simulink model "Simulink Model AC-DC Power Transmission"  (R2024a)
settings: Solver=VariableStepAuto  StartTime=0.0  StopTime=5  RelTol=1e-3
values from neighbouring files (symbols this model uses):
  C1 = 1e-3    (= 0.001)    [Parameters.m]
  Ka = Vdcref/2    [Parameters.m]
  kii1 = 2*3.14*fbwi*R1/Ka    [Parameters.m]
  kiw1 = kpw1/a1^2/taul1    [Parameters.m]
  kpi1 = 2*3.14*fbwi*L1/Ka    [Parameters.m]
  kpw1 = 2*C1/k1/a1/taul1    [Parameters.m]
  L1 = 5e-3    (= 0.005)    [Parameters.m]
  m = 0.848    [Parameters.m]
  R1 = 0.001    [Parameters.m]
  Rbat = (Vdcref/Pdc)*(Vbat-Vdcref)    [Parameters.m]
  tauf1 = 1/2/3.14/100    (= 0.0015923566879)    [Parameters.m]
  Vbat = 900    [Parameters.m]
  Vdcref = 400*sqrt(2)*2/(m*sqrt(3))    [Parameters.m]
  Vll = 400    [Parameters.m]
  w = 2*pi*f    (= 314.159265359)    [Parameters.m]
libraries: spsSeriesRLCBranchLib x9, spsIGBTDiodeLib x6, spsVoltageMeasurementLib x3, spsCurrentMeasurementLib x3, spsBreakerLib x1, spsDCVoltageSourceLib x1, spsTriangleGeneratorLib x1, spsThreePhaseBreakerLib x1, spsThreePhaseSourceLib x1, sps_lib x1
settings Model: SimulationMode=accelerator  Creator=akash  LastModifiedBy=Rhythm Shah
settings SolverCC: ZeroCrossAlgorithm=Adaptive
settings DebuggingCC: IgnoredZcDiagnostic=none

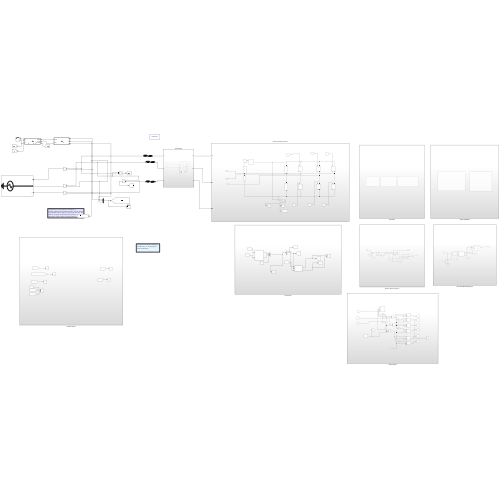
[thumbnail: Simulink's stored preview of the top-level diagram]
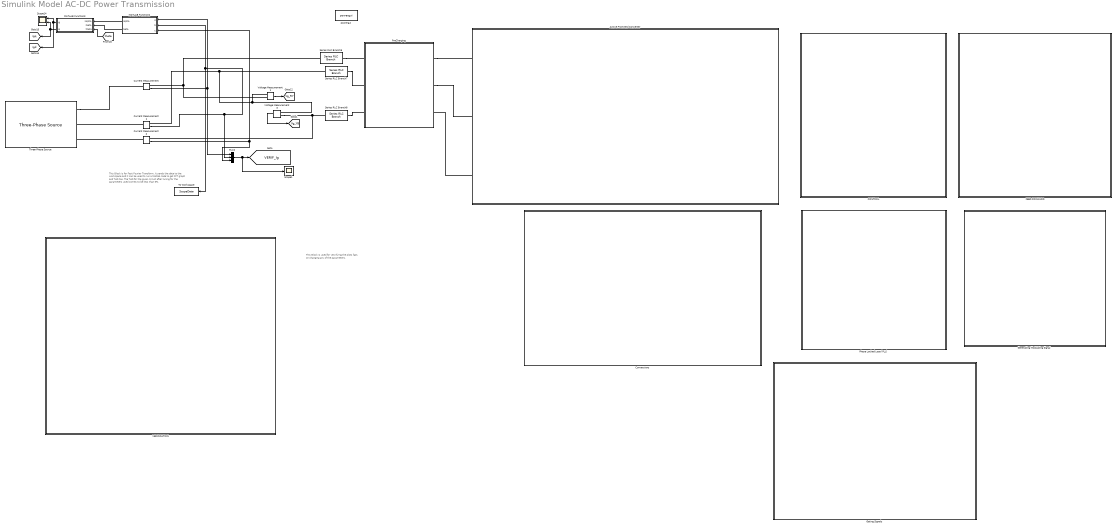
== system Simulink Model AC-DC Power Transmission ==
  note: This Block is used for veryifying
      | the plots fast, on changing any
      | of the parameters.
  note: This Block is for Fast Fourier Transform, it
      | sends the data to the workspace and it can be used to
      | run a Matlab code to get FFT graph and THD too. The
      | THD for the given circuit after tuning for the
      | parameters used comes to be less than 5%.
  Active Front End Converter : Subsystem
  CONTROL : Subsystem
  Conversions : Subsystem
  Current Measurement : spsCurrentMeasurementLib/Current Measurement  PhasorSimulation=off  OutputType=Complex  PSBequivalent=0
  Current Measurement1 : spsCurrentMeasurementLib/Current Measurement  PhasorSimulation=off  OutputType=Complex  PSBequivalent=0
  Current Measurement2 : spsCurrentMeasurementLib/Current Measurement  PhasorSimulation=off  OutputType=Complex  PSBequivalent=0
  FEED FORWARD : Subsystem
  Gating Signals : Subsystem
  Generating Modulating Signal : Subsystem
  MATLAB Function2 : MATLAB Function  TreatAsAtomicUnit=on
  MATLAB Function3 : MATLAB Function  TreatAsAtomicUnit=on
  Mux2 : Mux  Inputs=3
  Phase Locked Loop (PLL) : Subsystem
  PreCharging : Subsystem
  Scope1 : Scope
  Scope14 : Scope  NumInputPorts=2
  Series RLC Branch6 : spsSeriesRLCBranchLib/Series RLC Branch  LConnTagsString=__new0  RConnTagsString=__new0  BranchType=RL  Resistance=R1  Inductance=L1  SetiL0=off  InitialCurrent=0  Capacitance=1e-6  Setx0=off  InitialVoltage=0  Measurements=None
  Series RLC Branch7 : spsSeriesRLCBranchLib/Series RLC Branch  LConnTagsString=__new0  RConnTagsString=__new0  BranchType=RL  Resistance=R1  Inductance=L1  SetiL0=off  InitialCurrent=0  Capacitance=1e-6  Setx0=off  InitialVoltage=0  Measurements=None
  Series RLC Branch8 : spsSeriesRLCBranchLib/Series RLC Branch  LConnTagsString=__new0  RConnTagsString=__new0  BranchType=RL  Resistance=R1  Inductance=L1  SetiL0=off  InitialCurrent=0  Capacitance=1e-6  Setx0=off  InitialVoltage=0  Measurements=None
  Three-Phase Source : spsThreePhaseSourceLib/Three-Phase Source  InternalConnection=Yg  VoltagePhases=off  Voltage=Vll  PhaseAngle=0  Voltage_phases=[25e3 25e3 25e3]/sqrt(3)  PhaseAngles_phases=[0 -120 +120]  Frequency=50  NonIdealSource=off  SpecifyImpedance=off  Resistance=0  Inductance=0  ShortCircuitLevel=100e6  BaseVoltage=0  XRratio=7  BusType=swing  Pref=10e3  Qref=0  Prefabc=[10e3, 10e3, 10e3]  Qrefabc=[0, 0, 0]  Qmin=-inf  Qmax=inf
  To Workspace : ToWorkspace  VariableName=ScopeData  SaveFormat=Structure With Time  SampleTime=-1
  VERIFICATION : Subsystem
  Voltage Measurement1 : spsVoltageMeasurementLib/Voltage Measurement  PhasorSimulation=off  OutputType=Complex  PSBequivalent=0
  Voltage Measurement3 : spsVoltageMeasurementLib/Voltage Measurement  PhasorSimulation=off  OutputType=Complex  PSBequivalent=0
  powergui : sps_lib/powergui  Priority=1  SimulationMode=Continuous  SampleTime=50e-6  frequency=60  Iterations=50  frequencyindice=0  Pbase=100e6  ErrMax=1e-4  UnitsV=kV  UnitsW=MW  buscounter=0  FunctionMessages=off  echomessages=off  EnableUseOfTLC=off  CurrentSourceSwitches=off  DisableSnubberDevices=off  DisableRonSwitches=off  DisableVfSwitches=off  DisplayEquations=off  AutomaticDiscreteSolvers=off  SolverType=Tustin/Backward Euler (TBE)  Interpol=off  ExternalGateDelay=off  methode=off  Ts=100  x0status=blocks  SPID=on  SwTol=0  HookPort=off  NonlinearTolerance=1e-4  nMaxIteration=100  ContinueOnMaxIteration=off  RestoreLinks=warning  ResistiveCurrentMeasurement=off  Frange=[0:2:500]  Ylog=off  Xlog=on  ShowGrid=off  save=off  variable=ZData  structure=0  ZoomFFT=off  StartTime=0.0  cycles=1  DisplayStyle=1  fundamental=60  FreqAxis=off  MaxFrequency=1000  frequencyindicesteady=1  RmsSteady=1  display=off
  tag scope: VERIF_Ig=global, Vg_RY=global, Vg_YB=global, igd=global, igq=global
  wires:
  Current Measurement1/1 -> MATLAB Function2/2(b), To Workspace/1, Mux2/2
  Current Measurement/1 -> Mux2/1, MATLAB Function2/1(a)
  Current Measurement2/1 -> MATLAB Function2/3(c), Mux2/3
  Voltage Measurement1/1 -> [Vg_RY]
  Voltage Measurement3/1 -> [Vg_YB]
  Mux2/1 -> [VERIF_Ig], Scope1/1
  MATLAB Function3/2(iq) -> [igq], Scope14/2
  [theta] -> MATLAB Function3/3(theta)
  MATLAB Function2/2(beta) -> MATLAB Function3/2(ibeta)
  MATLAB Function2/1(alpha) -> MATLAB Function3/1(ialpha)
  MATLAB Function3/1(id) -> [igd], Scope14/1
  connections:
  Voltage Measurement3/LConn2 -- Current Measurement2/RConn1 -- Series RLC Branch8/RConn1
  Voltage Measurement1/LConn2 -- Current Measurement1/RConn1 -- Series RLC Branch7/RConn1 -- Voltage Measurement3/LConn1
  Voltage Measurement1/LConn1 -- Current Measurement/RConn1 -- Series RLC Branch6/RConn1
  Three-Phase Source/RConn1 -- Current Measurement/LConn1
  Current Measurement2/LConn1 -- Three-Phase Source/RConn3
  Current Measurement1/LConn1 -- Three-Phase Source/RConn2
  PreCharging/LConn1 -- Active Front End Converter/RConn1
  PreCharging/LConn2 -- Active Front End Converter/RConn2
  Series RLC Branch6/LConn1 -- PreCharging/RConn1
  Series RLC Branch7/LConn1 -- PreCharging/RConn2
  Active Front End Converter/RConn3 -- PreCharging/LConn3
  Series RLC Branch8/LConn1 -- PreCharging/RConn3

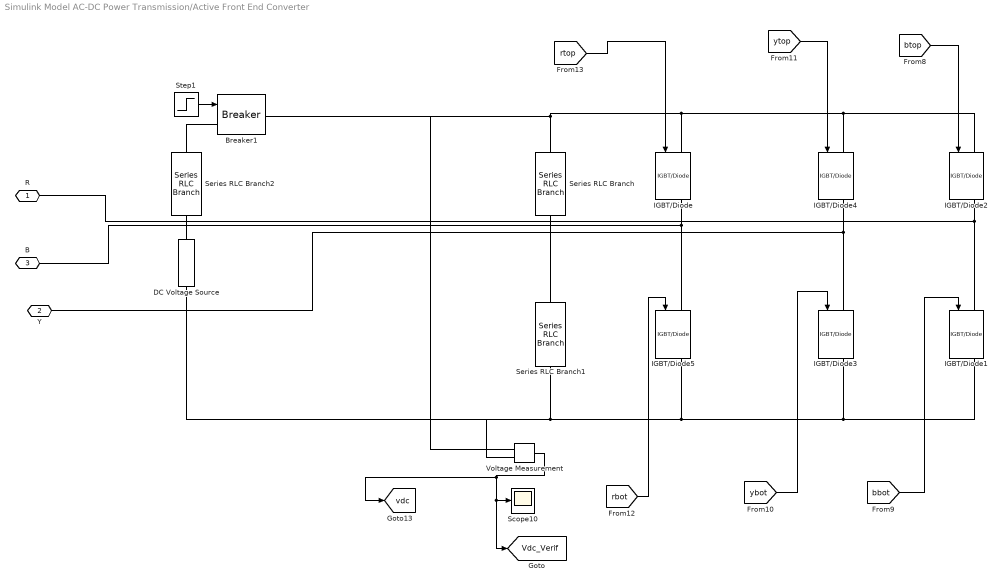
== system Simulink Model AC-DC Power Transmission/Active Front End Converter ==
  Breaker1 : spsBreakerLib/Breaker  InitialState=0  SwitchingTimes="[1/60  5/60]"  External=on  BreakerResistance=0.01  SnubberResistance=1e6  SnubberCapacitance=inf  Measurements=None  MoreParameters=on  NoBreakLoop=off
  DC Voltage Source : spsDCVoltageSourceLib/DC Voltage Source  Amplitude=Vbat  Measurements=None
  IGBT/Diode{,1..5} (6 alike) : spsIGBTDiodeLib/IGBT//Diode  Ron=1e-5  Rs=1e7  Cs=inf  Measurements=on
  Scope10 : Scope
  Series RLC Branch : spsSeriesRLCBranchLib/Series RLC Branch  LConnTagsString=__new0  RConnTagsString=__new0  BranchType=C  Resistance=0  Inductance=0  SetiL0=off  InitialCurrent=0  Capacitance=C1  Setx0=on  InitialVoltage=0  Measurements=None
  Series RLC Branch1 : spsSeriesRLCBranchLib/Series RLC Branch  LConnTagsString=__new0  RConnTagsString=__new0  BranchType=C  Resistance=0  Inductance=0  SetiL0=off  InitialCurrent=0  Capacitance=C1  Setx0=on  InitialVoltage=0  Measurements=None
  Series RLC Branch2 : spsSeriesRLCBranchLib/Series RLC Branch  LConnTagsString=__new0  RConnTagsString=__new0  BranchType=R  Resistance=Rbat  Inductance=0  SetiL0=off  InitialCurrent=0  Capacitance=1e-6  Setx0=off  InitialVoltage=0  Measurements=None
  Step1 : Step  Time=0.6  SampleTime=0
  Voltage Measurement : spsVoltageMeasurementLib/Voltage Measurement  PhasorSimulation=off  OutputType=Complex  PSBequivalent=0
  R : PMIOPort  Side=Right
  Y : PMIOPort  Port=2  Side=Right
  B : PMIOPort  Port=3  Side=Right
  tag scope: Vdc_Verif=global, vdc=global
  wires:
  [ybot] -> IGBT/Diode3/1
  [rtop] -> IGBT/Diode/1
  [bbot] -> IGBT/Diode1/1
  [ytop] -> IGBT/Diode4/1
  Step1/1 -> Breaker1/1
  [rbot] -> IGBT/Diode5/1
  [btop] -> IGBT/Diode2/1
  Voltage Measurement/1 -> [vdc], [Vdc_Verif], Scope10/1
  connections:
  IGBT/Diode4/RConn1 -- IGBT/Diode3/LConn1 -- Y/RConn1
  IGBT/Diode2/RConn1 -- IGBT/Diode1/LConn1 -- R/RConn1
  Breaker1/LConn1 -- Series RLC Branch2/LConn1
  IGBT/Diode3/RConn1 -- Series RLC Branch1/RConn1 -- DC Voltage Source/LConn1 -- Voltage Measurement/LConn2 -- IGBT/Diode5/RConn1 -- IGBT/Diode1/RConn1
  IGBT/Diode4/LConn1 -- IGBT/Diode/LConn1 -- Voltage Measurement/LConn1 -- Breaker1/RConn1 -- Series RLC Branch/LConn1 -- IGBT/Diode2/LConn1
  IGBT/Diode/RConn1 -- B/RConn1 -- IGBT/Diode5/LConn1
  DC Voltage Source/RConn1 -- Series RLC Branch2/RConn1
  Series RLC Branch1/LConn1 -- Series RLC Branch/RConn1

== system Simulink Model AC-DC Power Transmission/CONTROL ==
  Id Current control : Subsystem
  Iq Current Control : Subsystem
  Voltage control : Subsystem

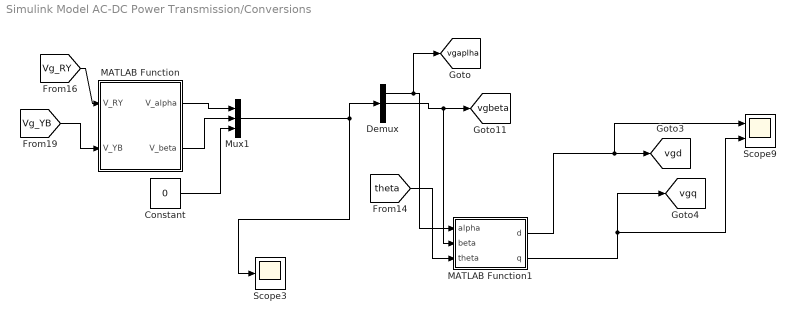
== system Simulink Model AC-DC Power Transmission/Conversions ==
  Constant : Constant  Value=0
  Demux : Demux  Outputs=3
  MATLAB Function : MATLAB Function  TreatAsAtomicUnit=on
  MATLAB Function1 : MATLAB Function  TreatAsAtomicUnit=on
  Mux1 : Mux  Inputs=3
  Scope3 : Scope
  Scope9 : Scope  NumInputPorts=2
  tag scope: vgaplha=global, vgbeta=global, vgd=global, vgq=global
  wires:
  Mux1/1 -> Scope3/1, Demux/1
  MATLAB Function/1(V_alpha) -> Mux1/1
  Demux/2 -> MATLAB Function1/2(beta), [vgbeta]
  Demux/1 -> MATLAB Function1/1(alpha), [vgaplha]
  MATLAB Function1/2(q) -> [vgq], Scope9/2
  [Vg_YB] -> MATLAB Function/2(V_YB)
  MATLAB Function1/1(d) -> Scope9/1, [vgd]
  [theta] -> MATLAB Function1/3(theta)
  MATLAB Function/2(V_beta) -> Mux1/2
  [Vg_RY] -> MATLAB Function/1(V_RY)
  Constant/1 -> Mux1/3

== system Simulink Model AC-DC Power Transmission/FEED FORWARD ==
  Id Feed Forward : Subsystem
  Iq Feed Forward : Subsystem

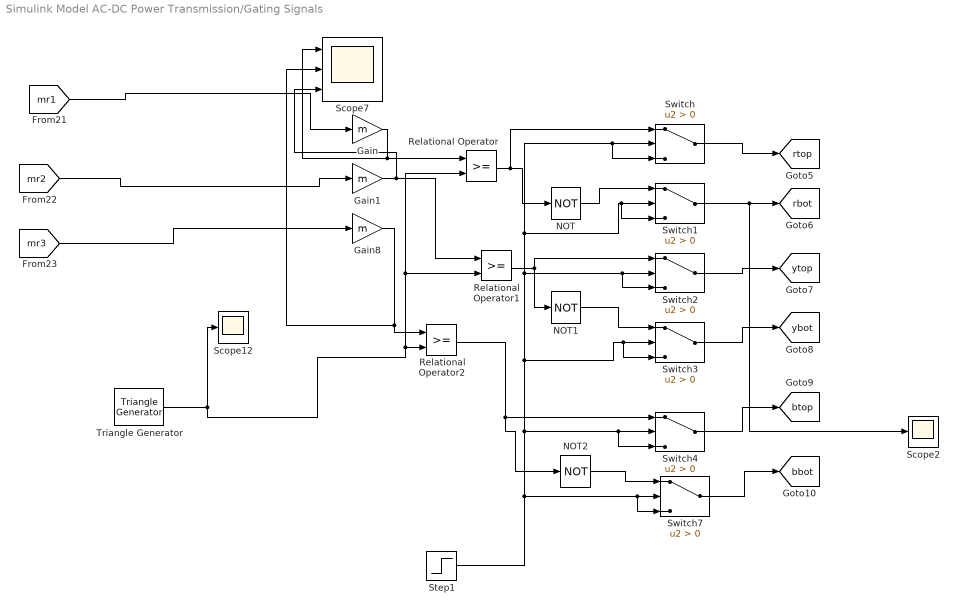
== system Simulink Model AC-DC Power Transmission/Gating Signals ==
  Gain : Gain  Gain=m
  Gain1 : Gain  Gain=m
  Gain8 : Gain  Gain=m
  NOT : Logic  Operator=NOT  IconShape=distinctive  AllPortsSameDT=off  OutDataTypeStr=boolean
  NOT1 : Logic  Operator=NOT  IconShape=distinctive  AllPortsSameDT=off  OutDataTypeStr=boolean
  NOT2 : Logic  Operator=NOT  IconShape=distinctive  AllPortsSameDT=off  OutDataTypeStr=boolean
  Relational Operator : RelationalOperator  OutDataTypeStr=boolean  RndMeth=Simplest  InputSameDT=off
  Relational Operator1 : RelationalOperator  OutDataTypeStr=boolean  RndMeth=Simplest  InputSameDT=off
  Relational Operator2 : RelationalOperator  OutDataTypeStr=boolean  RndMeth=Simplest  InputSameDT=off
  Scope12 : Scope
  Scope2 : Scope
  Scope7 : Scope  NumInputPorts=3
  Step1 : Step  SampleTime=0
  Switch{,1..4,7} (6 alike) : Switch  Criteria=u2 > Threshold  SaturateOnIntegerOverflow=off  InputSameDT=off
  Triangle Generator : spsTriangleGeneratorLib/Triangle Generator  Freq=5000  Phase=0  Ts=0
  tag scope: bbot=global, btop=global, rbot=global, rtop=global, ybot=global, ytop=global
  wires:
  NOT/1 -> Switch1/1
  [mr3] -> Gain8/1
  Switch1/1 -> Scope2/1, [rbot]
  Gain1/1 -> Relational Operator1/1, Scope7/3
  Gain/1 -> Relational Operator/1, Scope7/1
  Switch7/1 -> [bbot]
  NOT2/1 -> Switch7/1
  Triangle Generator/1 -> Relational Operator2/2, Relational Operator1/2, Relational Operator/2, Scope12/1
  Relational Operator1/1 -> Switch2/1, NOT1/1
  Relational Operator/1 -> Switch/1, NOT/1
  [mr1] -> Gain/1
  Switch2/1 -> [ytop]
  Step1/1 -> Switch7/3, Switch7/2, Switch4/3, Switch4/2, Switch3/3, Switch3/2, Switch1/3, Switch1/2, Switch/3, Switch/2, Switch2/3, Switch2/2
  Gain8/1 -> Scope7/2, Relational Operator2/1
  Relational Operator2/1 -> NOT2/1, Switch4/1
  [mr2] -> Gain1/1
  Switch3/1 -> [ybot]
  Switch/1 -> [rtop]
  Switch4/1 -> [btop]
  NOT1/1 -> Switch3/1

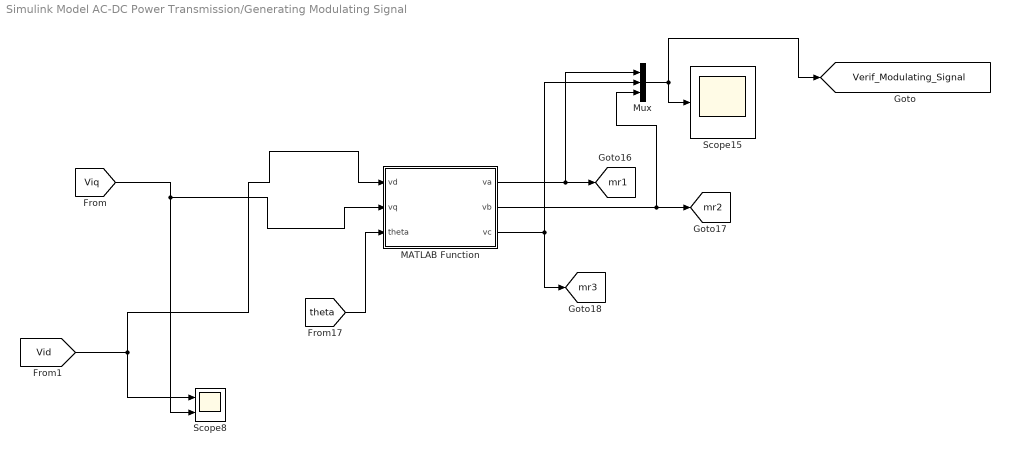
== system Simulink Model AC-DC Power Transmission/Generating Modulating Signal ==
  MATLAB Function : MATLAB Function  TreatAsAtomicUnit=on
  Mux : Mux  Inputs=3
  Scope15 : Scope
  Scope8 : Scope  NumInputPorts=2
  tag scope: Verif_Modulating_Signal=global, mr1=global, mr2=global, mr3=global
  wires:
  MATLAB Function/1(va) -> Mux/1, [mr1]
  MATLAB Function/2(vb) -> Mux/3, [mr2]
  [theta] -> MATLAB Function/3(theta)
  [Vid] -> MATLAB Function/1(vd), Scope8/1
  MATLAB Function/3(vc) -> Mux/2, [mr3]
  [Viq] -> Scope8/2, MATLAB Function/2(vq)
  Mux/1 -> [Verif_Modulating_Signal], Scope15/1

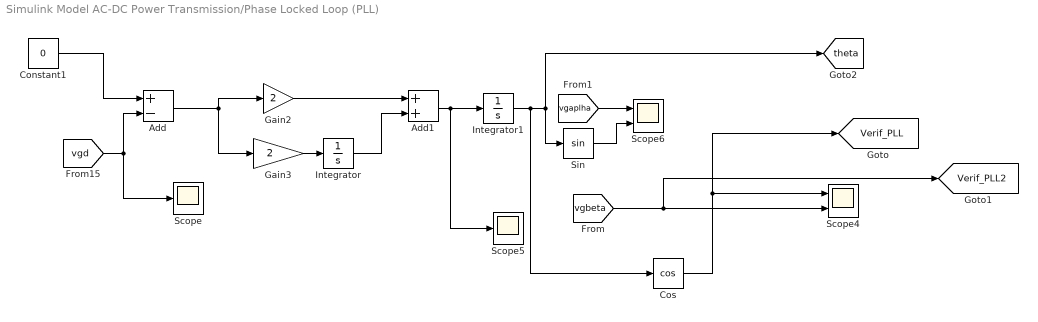
== system Simulink Model AC-DC Power Transmission/Phase Locked Loop (PLL) ==
  Add : Sum  Inputs=+-
  Add1 : Sum
  Constant1 : Constant  Value=0
  Cos : Trigonometry  Operator=cos
  Gain2 : Gain  Gain=2
  Gain3 : Gain  Gain=2
  Integrator : Integrator
  Integrator1 : Integrator
  Scope : Scope
  Scope4 : Scope  NumInputPorts=2
  Scope5 : Scope
  Scope6 : Scope  NumInputPorts=2
  Sin : Trigonometry
  tag scope: Verif_PLL2=global, Verif_PLL=global, theta=global
  wires:
  Constant1/1 -> Add/1
  [vgbeta] -> [Verif_PLL2], Scope4/2
  Integrator/1 -> Add1/2
  Gain3/1 -> Integrator/1
  [vgd] -> Scope/1, Add/2
  Sin/1 -> Scope6/2
  Gain2/1 -> Add1/1
  Integrator1/1 -> Cos/1, [theta], Sin/1
  Add/1 -> Gain3/1, Gain2/1
  Add1/1 -> Scope5/1, Integrator1/1
  Cos/1 -> [Verif_PLL], Scope4/1
  [vgaplha] -> Scope6/1

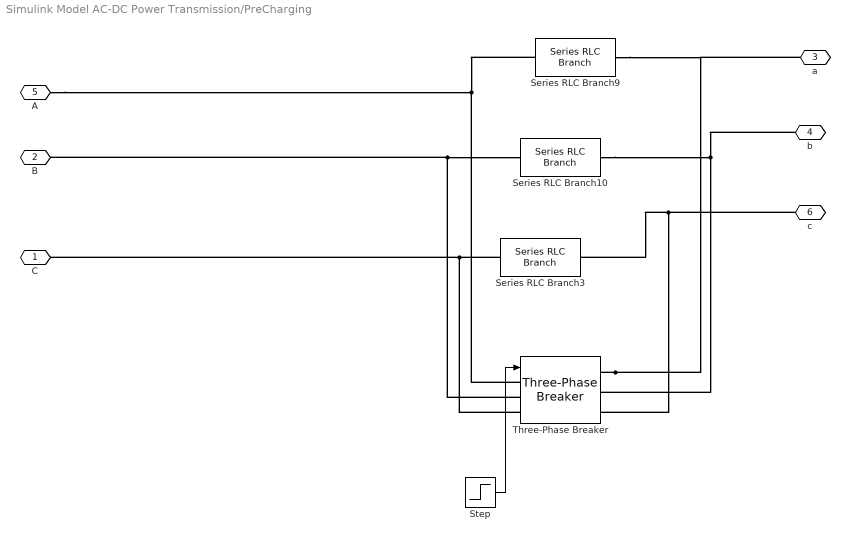
== system Simulink Model AC-DC Power Transmission/PreCharging ==
  Series RLC Branch10 : spsSeriesRLCBranchLib/Series RLC Branch  LConnTagsString=__new0  RConnTagsString=__new0  BranchType=R  Resistance=50  Inductance=1e-3  SetiL0=off  InitialCurrent=0  Capacitance=1e-6  Setx0=off  InitialVoltage=0  Measurements=None
  Series RLC Branch3 : spsSeriesRLCBranchLib/Series RLC Branch  LConnTagsString=__new0  RConnTagsString=__new0  BranchType=R  Resistance=50  Inductance=1e-3  SetiL0=off  InitialCurrent=0  Capacitance=1e-6  Setx0=off  InitialVoltage=0  Measurements=None
  Series RLC Branch9 : spsSeriesRLCBranchLib/Series RLC Branch  LConnTagsString=__new0  RConnTagsString=__new0  BranchType=R  Resistance=50  Inductance=1e-3  SetiL0=off  InitialCurrent=0  Capacitance=1e-6  Setx0=off  InitialVoltage=0  Measurements=None
  Step : Step  Time=0.6  SampleTime=0
  Three-Phase Breaker : spsThreePhaseBreakerLib/Three-Phase Breaker  InitialState=open  SwitchA=on  SwitchB=on  SwitchC=on  SwitchTimes="[1/60  5/60]"  External=on  BreakerResistance=0.01  SnubberResistance=1e6  SnubberCapacitance=inf  Measurements=None
  C : PMIOPort  Side=Left
  B : PMIOPort  Port=2  Side=Left
  a : PMIOPort  Port=3  Side=Right
  b : PMIOPort  Port=4  Side=Right
  A : PMIOPort  Port=5  Side=Left
  c : PMIOPort  Port=6  Side=Right
  wires:
  Step/1 -> Three-Phase Breaker/1
  connections:
  Three-Phase Breaker/RConn1 -- a/RConn1 -- Series RLC Branch9/RConn1
  c/RConn1 -- Three-Phase Breaker/RConn3 -- Series RLC Branch3/RConn1
  Three-Phase Breaker/LConn3 -- C/RConn1 -- Series RLC Branch3/LConn1
  Series RLC Branch10/RConn1 -- b/RConn1 -- Three-Phase Breaker/RConn2
  Three-Phase Breaker/LConn2 -- Series RLC Branch10/LConn1 -- B/RConn1
  Series RLC Branch9/LConn1 -- Three-Phase Breaker/LConn1 -- A/RConn1

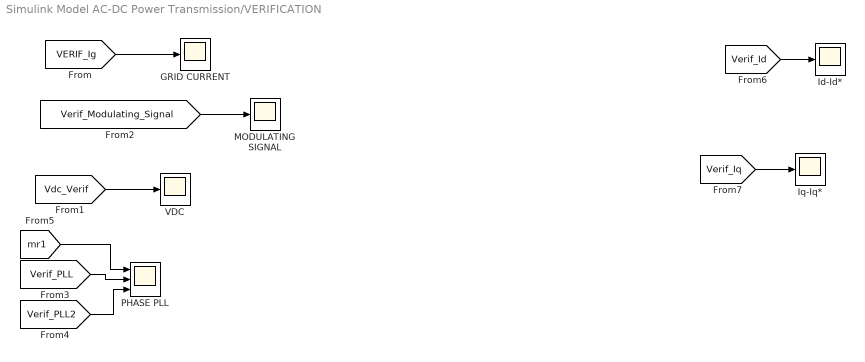
== system Simulink Model AC-DC Power Transmission/VERIFICATION ==
  GRID CURRENT : Scope
  Id-Id* : Scope
  Iq-Iq* : Scope
  MODULATING SIGNAL : Scope
  PHASE PLL : Scope  NumInputPorts=3
  VDC : Scope
  wires:
  [VERIF_Ig] -> GRID CURRENT/1
  [Verif_Modulating_Signal] -> MODULATING SIGNAL/1
  [Vdc_Verif] -> VDC/1
  [Verif_PLL] -> PHASE PLL/2
  [Verif_PLL2] -> PHASE PLL/3
  [mr1] -> PHASE PLL/1
  [Verif_Id] -> Id-Id*/1
  [Verif_Iq] -> Iq-Iq*/1

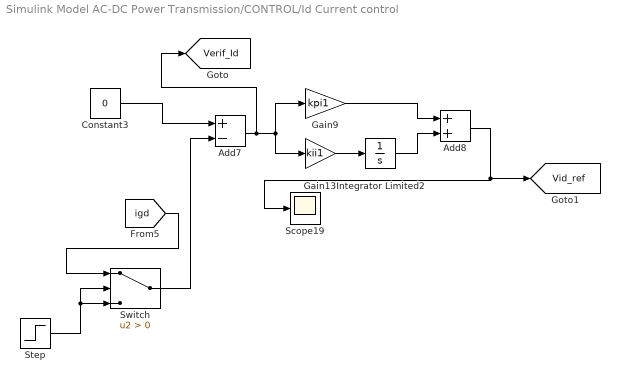
== system Simulink Model AC-DC Power Transmission/CONTROL/Id Current control ==
  Add7 : Sum  Inputs=+-
  Add8 : Sum
  Constant3 : Constant  Value=0
  Gain13 : Gain  Gain=kii1
  Gain9 : Gain  Gain=kpi1
  Integrator Limited2 : Integrator  LimitOutput=on  UpperSaturationLimit=1  LowerSaturationLimit=-1
  Scope19 : Scope
  Step : Step  SampleTime=0
  Switch : Switch  Criteria=u2 > Threshold  SaturateOnIntegerOverflow=off  InputSameDT=off
  tag scope: Verif_Id=global, Vid_ref=global
  wires:
  Gain13/1 -> Integrator Limited2/1
  Integrator Limited2/1 -> Add8/2
  Constant3/1 -> Add7/1
  Gain9/1 -> Add8/1
  Add7/1 -> [Verif_Id], Gain9/1, Gain13/1
  Add8/1 -> Scope19/1, [Vid_ref]
  Step/1 -> Switch/3, Switch/2
  Switch/1 -> Add7/2
  [igd] -> Switch/1

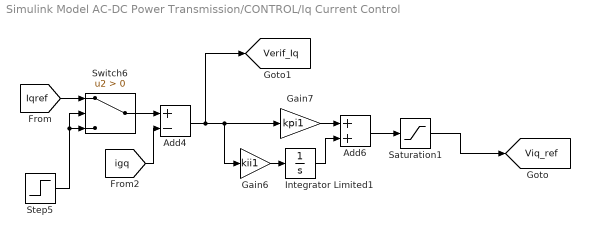
== system Simulink Model AC-DC Power Transmission/CONTROL/Iq Current Control ==
  Add4 : Sum  Inputs=+-
  Add6 : Sum
  Gain6 : Gain  Gain=kii1
  Gain7 : Gain  Gain=kpi1
  Integrator Limited1 : Integrator  LimitOutput=on  UpperSaturationLimit=1  LowerSaturationLimit=-1
  Saturation1 : Saturate  UpperLimit=1  LowerLimit=-1
  Step5 : Step  SampleTime=0
  Switch6 : Switch  Criteria=u2 > Threshold  SaturateOnIntegerOverflow=off  InputSameDT=off
  tag scope: Verif_Iq=global, Viq_ref=global
  wires:
  Step5/1 -> Switch6/3, Switch6/2
  Integrator Limited1/1 -> Add6/2
  [igq] -> Add4/2
  Gain7/1 -> Add6/1
  Add4/1 -> [Verif_Iq], Gain6/1, Gain7/1
  Switch6/1 -> Add4/1
  Add6/1 -> Saturation1/1
  Gain6/1 -> Integrator Limited1/1
  [Iqref] -> Switch6/1
  Saturation1/1 -> [Viq_ref]

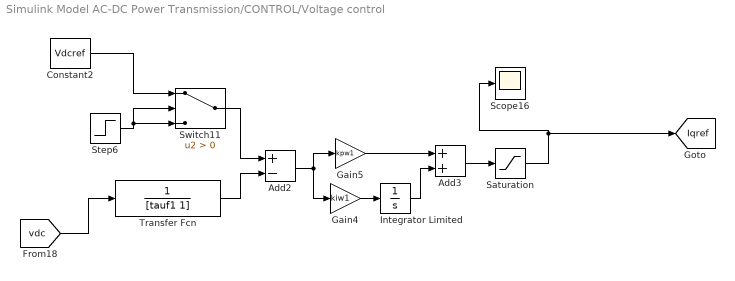
== system Simulink Model AC-DC Power Transmission/CONTROL/Voltage control ==
  Add2 : Sum  Inputs=+-
  Add3 : Sum
  Constant2 : Constant  Value=Vdcref
  Gain4 : Gain  Gain=kiw1
  Gain5 : Gain  Gain=kpw1
  Integrator Limited : Integrator  LimitOutput=on  UpperSaturationLimit=25  LowerSaturationLimit=-25
  Saturation : Saturate  UpperLimit=25  LowerLimit=-25
  Scope16 : Scope
  Step6 : Step  Time=1.5  SampleTime=0
  Switch11 : Switch  Criteria=u2 > Threshold  SaturateOnIntegerOverflow=off  InputSameDT=off
  Transfer Fcn : TransferFcn  Denominator=[tauf1 1]
  tag scope: Iqref=global
  wires:
  Transfer Fcn/1 -> Add2/2
  Integrator Limited/1 -> Add3/2
  Switch11/1 -> Add2/1
  Gain4/1 -> Integrator Limited/1
  [vdc] -> Transfer Fcn/1
  Constant2/1 -> Switch11/1
  Gain5/1 -> Add3/1
  Step6/1 -> Switch11/2, Switch11/3
  Add3/1 -> Saturation/1
  Add2/1 -> Gain4/1, Gain5/1
  Saturation/1 -> [Iqref], Scope16/1

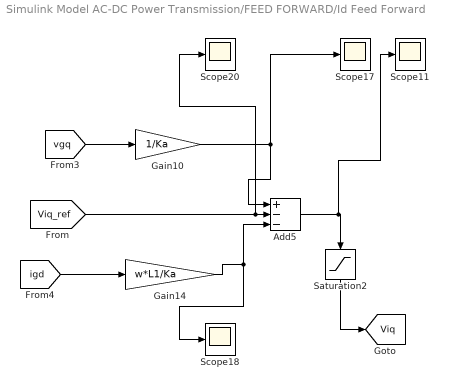
== system Simulink Model AC-DC Power Transmission/FEED FORWARD/Id Feed Forward ==
  Add5 : Sum  Inputs=+--
  Gain10 : Gain  Gain=1/Ka
  Gain14 : Gain  Gain=w*L1/Ka
  Saturation2 : Saturate  UpperLimit=1  LowerLimit=-1
  Scope{11,17..18,20} (4 alike) : Scope
  tag scope: Viq=global
  wires:
  [vgq] -> Gain10/1
  Add5/1 -> Scope11/1, Saturation2/1
  [Viq_ref] -> Scope20/1, Add5/2
  Gain14/1 -> Scope18/1, Add5/3
  [igd] -> Gain14/1
  Saturation2/1 -> [Viq]
  Gain10/1 -> Add5/1, Scope17/1

== system Simulink Model AC-DC Power Transmission/FEED FORWARD/Iq Feed Forward ==
  Add9 : Sum  Inputs=+-+
  Gain11 : Gain  Gain=1/Ka
  Gain12 : Gain  Gain=w*L1/Ka
  Saturation3 : Saturate  UpperLimit=1  LowerLimit=-1
  tag scope: Vid=global
  wires:
  Gain12/1 -> Add9/3
  Saturation3/1 -> [Vid]
  [Vid_ref] -> Add9/2
  [vgd] -> Gain11/1
  Gain11/1 -> Add9/1
  Add9/1 -> Saturation3/1
  [igq] -> Gain12/1

== matlab function Simulink Model AC-DC Power Transmission/Conversions/MATLAB Function1 ==
  data: alpha input; d output; beta input; theta input; q output
function[d,q]=alphabeta_to_dq(alpha, beta, theta)

    d=alpha*cos(theta)+beta*sin(theta);
    q=-alpha*sin(theta)+beta*cos(theta);
end

== matlab function Simulink Model AC-DC Power Transmission/Conversions/MATLAB Function ==
  data: V_RY input; V_alpha output; V_YB input; V_beta output
function [V_alpha , V_beta] = fcn(V_RY,V_YB)
% Convert line-to-line voltages to phase voltages
    V_R = V_RY / sqrt(3) * exp(-1i * pi / 6); % -30 degrees phase shift
    V_Y = V_YB / sqrt(3) * exp(-1i * pi / 6); % -30 degrees phase shift
    
    % Assume balanced system, so V_B = -(V_R + V_Y)
    V_B = -(V_R + V_Y);
    
    % Extract real parts for Clarke Transformation (phase voltages)
    V_R = real(V_R);
    V_Y = real(V_Y);
    V_B = real(V_B);
    
    % Apply Clarke Transform to get alpha-beta components
    V_alph = (2/3) * (V_R - 0.5 * V_Y - 0.5 * V_B);
    V_bet = (2/3) * (sqrt(3)/2 * (V_Y - V_B));
V_alpha = V_alph;
V_beta = V_bet;
end

== matlab function Simulink Model AC-DC Power Transmission/MATLAB Function2 ==
  data: a input; alpha output; b input; c input; beta output
function [alpha,beta]=abctoalphabeta(a,b,c)

    alpha=(2/3)*(a-0.5*b-0.5*c);
    beta=(2/3)*(sqrt(3)/2*(b-c));
end

== matlab function Simulink Model AC-DC Power Transmission/MATLAB Function3 ==
  data: ialpha input; id output; ibeta input; theta input; iq output
function [id,iq]=alphabeta_to_dq(ialpha,ibeta,theta)
    
    id=ialpha*cos(theta)+ibeta*sin(theta);
    iq=-ialpha*sin(theta)+ibeta*cos(theta);
end

== matlab function Simulink Model AC-DC Power Transmission/Generating Modulating Signal/MATLAB Function ==
  data: vd input; va output; vq input; theta input; vb output; vc output
function [va,vb,vc] = dq_to_abc(vd,vq,theta)

    valpha=vd*cos(theta)-vq*sin(theta);
    vbeta=vd*sin(theta)+vq*cos(theta);

    va=valpha;
    vb=-0.5*valpha+(sqrt(3)/2)*vbeta;
    vc=-0.5*valpha-(sqrt(3)/2)*vbeta;
end
